simulink model "oldSlice"  (R2021a)
settings: Solver=VariableStepAuto  StartTime=0.0  StopTime=10.0  RelTol=1e-3
libraries: hdlsllib x5, simulink x5
settings Model: Creator=sbetu  LastModifiedBy=sbetu

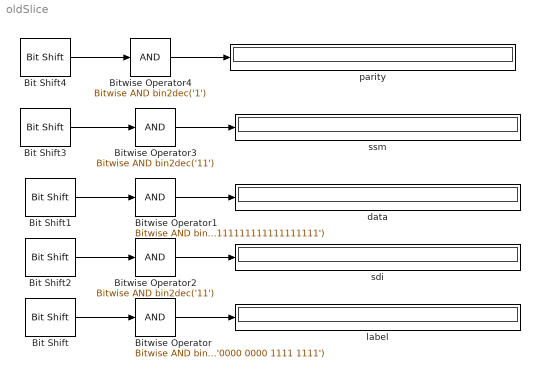
== system oldSlice ==
  Bit Shift : hdlsllib/Logic and Bit Operations/Bit Shift  mode=Shift Right Logical  N=1
  Bit Shift1 : hdlsllib/Logic and Bit Operations/Bit Shift  mode=Shift Right Logical  N=11
  Bit Shift2 : hdlsllib/Logic and Bit Operations/Bit Shift  mode=Shift Right Logical  N=9
  Bit Shift3 : hdlsllib/Logic and Bit Operations/Bit Shift  mode=Shift Right Logical  N=30
  Bit Shift4 : hdlsllib/Logic and Bit Operations/Bit Shift  mode=Shift Right Logical  N=32
  Bitwise Operator : simulink/Logic and Bit Operations/Bitwise Operator  logicop=AND  UseBitMask=on  BitMask=bin2dec('0000 0000 1111 1111')  BitMaskRealWorld=Stored Integer
  Bitwise Operator1 : simulink/Logic and Bit Operations/Bitwise Operator  logicop=AND  UseBitMask=on  BitMask=bin2dec('1111111111111111111')  BitMaskRealWorld=Stored Integer
  Bitwise Operator2 : simulink/Logic and Bit Operations/Bitwise Operator  logicop=AND  UseBitMask=on  BitMask=bin2dec('11')  BitMaskRealWorld=Stored Integer
  Bitwise Operator3 : simulink/Logic and Bit Operations/Bitwise Operator  logicop=AND  UseBitMask=on  BitMask=bin2dec('11')  BitMaskRealWorld=Stored Integer
  Bitwise Operator4 : simulink/Logic and Bit Operations/Bitwise Operator  logicop=AND  UseBitMask=on  BitMask=bin2dec('1')  BitMaskRealWorld=Stored Integer
  data : Display
      settings: Format=binary (Stored Integer)
  label : Display
      settings: Format=binary (Stored Integer)
  parity : Display
      settings: Format=binary (Stored Integer)
  sdi : Display
      settings: Format=binary (Stored Integer)
  ssm : Display
      settings: Format=binary (Stored Integer)
  wires:
  Bit Shift4/1 -> Bitwise Operator4/1
  Bitwise Operator4/1 -> parity/1
  Bitwise Operator/1 -> label/1
  Bit Shift/1 -> Bitwise Operator/1
  Bitwise Operator2/1 -> sdi/1
  Bit Shift2/1 -> Bitwise Operator2/1
  Bitwise Operator3/1 -> ssm/1
  ? -> Bit Shift4/1
  Bit Shift1/1 -> Bitwise Operator1/1
  ? -> Bit Shift1/1
  ? -> Bit Shift3/1
  Bitwise Operator1/1 -> data/1
  Bit Shift3/1 -> Bitwise Operator3/1
  ? -> Bit Shift/1
  ? -> Bit Shift2/1
